simulink model "ControlSystemCrustCrawler"  (R2020b)
settings: Solver=VariableStepAuto  StartTime=0.0  StopTime=10.0  RelTol=1e-3
model workspace: external: MATLAB File C:\Users\soren\Documents\MATLAB\FinalAss_DataFile5.m (data not in the file)
undefined symbols (not defined in the file or in its folder): smiData, X, Y, Z
libraries: sm_lib x109, nesl_utility x20, simulink_extras x4, pid_lib x3
(part 3 of 3)

== matlab function ControlSystemCrustCrawler/ComputedTorqueCG ==
  data: thetaCurrent input; ComputeCG output; dthetaCurrent input
function ComputeCG = Compute(thetaCurrent, dthetaCurrent)

theta1 = thetaCurrent(1);
theta2 = thetaCurrent(2);
theta3 = thetaCurrent(3);
theta4 = thetaCurrent(4);
dtheta1 = dthetaCurrent(1);
dtheta2 = dthetaCurrent(2);
dtheta3 = dthetaCurrent(3);
dtheta4 = dthetaCurrent(4);

CG1 = 0.0006*dtheta1*dtheta4*cos(theta4) - 0.0083*dtheta1*dtheta3*sin(theta3) - 0.0017*dtheta1*dtheta4*sin(theta4) - 0.0006*dtheta1*dtheta2*cos(2*theta2 + 2*theta3 + 2*theta4) - 0.0006*dtheta1*dtheta3*cos(2*theta2 + 2*theta3 + 2*theta4) - 0.0006*dtheta1*dtheta4*cos(2*theta2 + 2*theta3 + 2*theta4) - 0.0001*dtheta1*dtheta2*cos(2.0*theta2 + theta3) + 0.0007*dtheta1*dtheta2*sin(2*theta2 + 2*theta3 + 2*theta4) + 0.0007*dtheta1*dtheta3*sin(2*theta2 + 2*theta3 + 2*theta4) + 0.0007*dtheta1*dtheta4*sin(2*theta2 + 2*theta3 + 2*theta4) + 0.0165*dtheta1*dtheta2*sin(2.0*theta2 + theta3) + 0.0083*dtheta1*dtheta3*sin(2.0*theta2 + theta3) - 0.0013*dtheta1*dtheta2*cos(2.0*theta2 + 2.0*theta3 + theta4) - 0.0013*dtheta1*dtheta3*cos(2.0*theta2 + 2.0*theta3 + theta4) - 0.0006*dtheta1*dtheta4*cos(2.0*theta2 + 2.0*theta3 + theta4) + 0.0033*dtheta1*dtheta2*sin(2.0*theta2 + 2.0*theta3 + theta4) + 0.0033*dtheta1*dtheta3*sin(2.0*theta2 + 2.0*theta3 + theta4) + 0.0017*dtheta1*dtheta4*sin(2.0*theta2 + 2.0*theta3 + theta4) - 0.0001*dtheta1*dtheta2*cos(2.0*theta2) + 0.0052*dtheta1*dtheta2*sin(2*theta2 + 2*theta3) + 0.0052*dtheta1*dtheta3*sin(2*theta2 + 2*theta3) + 0.0233*dtheta1*dtheta2*sin(2.0*theta2) + 0.0010*dtheta1*dtheta3*cos(theta3 + theta4) + 0.0010*dtheta1*dtheta4*cos(theta3 + theta4) - 0.0025*dtheta1*dtheta3*sin(theta3 + theta4) - 0.0025*dtheta1*dtheta4*sin(theta3 + theta4) - 0.0020*dtheta1*dtheta2*cos(2.0*theta2 + theta3 + theta4) - 0.0010*dtheta1*dtheta3*cos(2.0*theta2 + theta3 + theta4) - 0.0010*dtheta1*dtheta4*cos(2.0*theta2 + theta3 + theta4) + 0.0050*dtheta1*dtheta2*sin(2.0*theta2 + theta3 + theta4) + 0.0025*dtheta1*dtheta3*sin(2.0*theta2 + theta3 + theta4) + 0.0025*dtheta1*dtheta4*sin(2.0*theta2 + theta3 + theta4);
CG2 = 0.3683*cos(theta2 + theta3 + 1.5636) + 0.1190*cos(theta2 + theta3 + theta4 + 1.1991) + 1.0545*cos(theta2 + 1.5686) - 0.0083*dtheta3^2*sin(theta3) - 0.0017*dtheta4^2*sin(theta4) + 0.0003*dtheta1^2*cos(2*theta2 + 2*theta3 + 2*theta4) + 0.0001*dtheta1^2*cos(2.0*theta2 + theta3) - 0.0003*dtheta1^2*sin(2*theta2 + 2*theta3 + 2*theta4) - 0.0083*dtheta1^2*sin(2.0*theta2 + theta3) + 0.0006*dtheta1^2*cos(2.0*theta2 + 2.0*theta3 + theta4) - 0.0017*dtheta1^2*sin(2.0*theta2 + 2.0*theta3 + theta4) + 0.0001*dtheta1^2*cos(2.0*theta2) - 0.0026*dtheta1^2*sin(2*theta2 + 2*theta3) - 0.0116*dtheta1^2*sin(2.0*theta2) + 0.0010*dtheta3^2*cos(theta3 + theta4) + 0.0010*dtheta4^2*cos(theta3 + theta4) - 0.0025*dtheta3^2*sin(theta3 + theta4) - 0.0025*dtheta4^2*sin(theta3 + theta4) + 0.0010*dtheta1^2*cos(2.0*theta2 + theta3 + theta4) - 0.0025*dtheta1^2*sin(2.0*theta2 + theta3 + theta4) + 0.0006*dtheta4^2*cos(theta4) + 0.0001*dtheta2*dtheta3*cos(theta3) + 0.0013*dtheta2*dtheta4*cos(theta4) + 0.0013*dtheta3*dtheta4*cos(theta4) - 0.0165*dtheta2*dtheta3*sin(theta3) - 0.0033*dtheta2*dtheta4*sin(theta4) - 0.0033*dtheta3*dtheta4*sin(theta4) + 0.0020*dtheta2*dtheta3*cos(theta3 + theta4) + 0.0020*dtheta2*dtheta4*cos(theta3 + theta4) + 0.0020*dtheta3*dtheta4*cos(theta3 + theta4) - 0.0050*dtheta2*dtheta3*sin(theta3 + theta4) - 0.0050*dtheta2*dtheta4*sin(theta3 + theta4) - 0.0050*dtheta3*dtheta4*sin(theta3 + theta4);
CG3 = 0.3683*cos(theta2 + theta3 + 1.5636) + 0.1190*cos(theta2 + theta3 + theta4 + 1.1991) + 0.0041*dtheta1^2*sin(theta3) + 0.0083*dtheta2^2*sin(theta3) - 0.0017*dtheta4^2*sin(theta4) + 0.0003*dtheta1^2*cos(2*theta2 + 2*theta3 + 2*theta4) - 0.0003*dtheta1^2*sin(2*theta2 + 2*theta3 + 2*theta4) - 0.0041*dtheta1^2*sin(2.0*theta2 + theta3) + 0.0006*dtheta1^2*cos(2.0*theta2 + 2.0*theta3 + theta4) - 0.0017*dtheta1^2*sin(2.0*theta2 + 2.0*theta3 + theta4) - 0.0026*dtheta1^2*sin(2*theta2 + 2*theta3) - 0.0005*dtheta1^2*cos(theta3 + theta4) - 0.0010*dtheta2^2*cos(theta3 + theta4) + 0.0012*dtheta1^2*sin(theta3 + theta4) + 0.0025*dtheta2^2*sin(theta3 + theta4) + 0.0005*dtheta1^2*cos(2.0*theta2 + theta3 + theta4) - 0.0012*dtheta1^2*sin(2.0*theta2 + theta3 + theta4) - 0.0001*dtheta2^2*cos(theta3) + 0.0006*dtheta4^2*cos(theta4) + 0.0013*dtheta2*dtheta4*cos(theta4) + 0.0013*dtheta3*dtheta4*cos(theta4) - 0.0033*dtheta2*dtheta4*sin(theta4) - 0.0033*dtheta3*dtheta4*sin(theta4);
CG4 = 0.1190*cos(theta2 + theta3 + theta4 + 1.1991) + 0.0008*dtheta1^2*sin(theta4) + 0.0017*dtheta2^2*sin(theta4) + 0.0017*dtheta3^2*sin(theta4) + 0.0003*dtheta1^2*cos(2*theta2 + 2*theta3 + 2*theta4) - 0.0003*dtheta1^2*sin(2*theta2 + 2*theta3 + 2*theta4) + 0.0003*dtheta1^2*cos(2.0*theta2 + 2.0*theta3 + theta4) - 0.0008*dtheta1^2*sin(2.0*theta2 + 2.0*theta3 + theta4) - 0.0005*dtheta1^2*cos(theta3 + theta4) - 0.0010*dtheta2^2*cos(theta3 + theta4) + 0.0012*dtheta1^2*sin(theta3 + theta4) + 0.0025*dtheta2^2*sin(theta3 + theta4) + 0.0005*dtheta1^2*cos(2.0*theta2 + theta3 + theta4) - 0.0012*dtheta1^2*sin(2.0*theta2 + theta3 + theta4) - 0.0003*dtheta1^2*cos(theta4) - 0.0006*dtheta2^2*cos(theta4) - 0.0006*dtheta3^2*cos(theta4) - 0.0013*dtheta2*dtheta3*cos(theta4) + 0.0033*dtheta2*dtheta3*sin(theta4);


ComputeCG = [CG1; CG2; CG3; CG4]
